simulink model "systema"  (Simulink 7.4)
settings: Solver=ode1  StartTime=0.0  StopTime=1  FixedStep=0.01  RelTol=1e-3
libraries: simulink x7, instrumentlib x2
CloseFcn:
  | rtwprivate ssgencode ModelCloseRequest systema
settings Model: Creator=L503823  LastModifiedBy=tweeter  BufferReuse=off
settings DataIOCC: SignalLoggingName=sigsOut
settings OptimizationCC: OptimizeBlockIOStorage=off  BufferReuse=off  EnforceIntegerDowncast=off  ExpressionFolding=off  FoldNonRolledExpr=off  LocalBlockOutputs=off  InitFltsAndDblsToZero=on
settings DebuggingCC: SaveWithParameterizedLinksMsg=none  SignalResolutionControl=TryResolveAllWithWarning  SolverPrmCheckMsg=none  MultiTaskDSMMsg=warning  MultiTaskCondExecSysMsg=none  StrictBusMsg=ErrorLevel1
settings HardwareCC: TargetUnknown=on
settings RTWCC: IncludeERTFirstTime=on
settings CodeAppCC: IgnoreCustomStorageClasses=off
settings GRTTargetCC: TargetFcnLib=ansi_tfl_tmw.mat  ModelReferenceCompliant=off  MatFileLogging=off

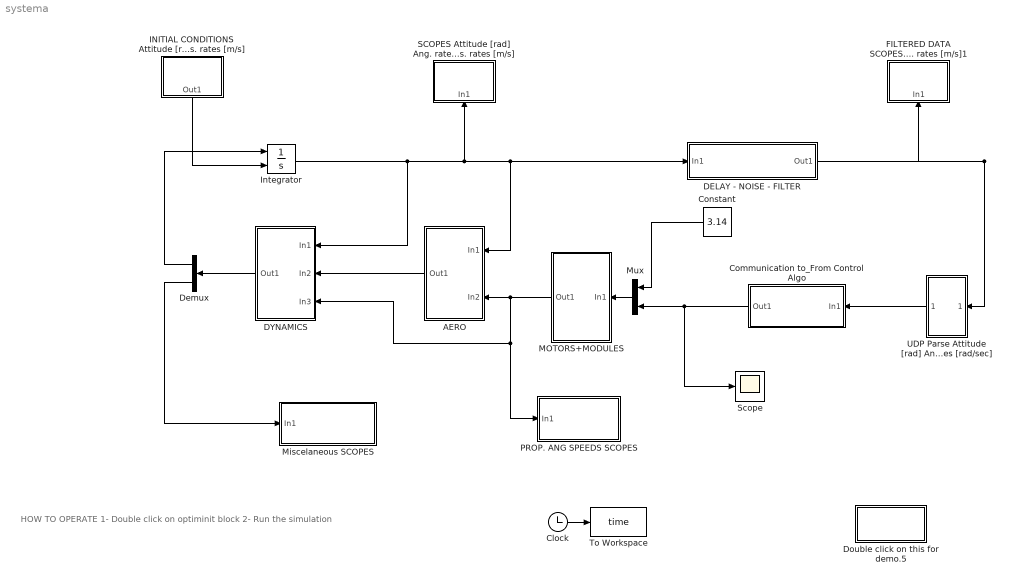
== system systema ==
  note: HOW TO OPERATE
      | 1- Double click on optiminit block
      | 2- Run the simulation
  AERO : Subsystem
  Clock : Clock
      settings: Decimation=10
  Communication to_From Control Algo : Subsystem  TreatAsAtomicUnit=on  SystemSampleTime=.01
  Constant : Constant  Value=3.14  OutDataTypeMode=double  OutDataType=fixdt(1, 16)  OutScaling=2^0  OutDataTypeStr=double  SampleTime=-1
  DELAY - NOISE - FILTER : Subsystem
  DYNAMICS : Subsystem
  Demux : Demux  Outputs=2
  Double click on this for demo.5 : Subsystem
      settings: OpenFcn=optsiminit
      mask Display: disp('optsiminit')
  FILTERED DATA SCOPES Attitude [rad] Ang. rates [rad/sec] position [m] Pos. rates [m/s]1 : Subsystem
  "INITIAL CONDITIONS Attitude [rad] Ang. rates [rad/sec] position [m] Pos. rates [m/s] " : Subsystem
  Integrator : Integrator  InitialConditionSource=external
  MOTORS+MODULES : Subsystem
  Miscelaneous SCOPES : Subsystem
  Mux : Mux  Inputs=2
  PROP. ANG SPEEDS SCOPES : Subsystem
  SCOPES Attitude [rad] Ang. rates [rad/sec] position [m] Pos. rates [m/s] : Subsystem
  Scope : Scope
      settings: YMin=-7.5e+06  YMax=1.25e+07  SaveName=ScopeData11
  To Workspace : ToWorkspace  VariableName=time  SampleTime=-1  SaveFormat=Array
  UDP Parse Attitude [rad] Ang. rates [rad/sec] : Subsystem  TreatAsAtomicUnit=on  SystemSampleTime=.01
  wires:
  Integrator/1 -> DYNAMICS/1(In1), AERO/1(In1), DELAY - NOISE - FILTER/1(In1), SCOPES Attitude [rad] Ang. rates [rad/sec] position [m] Pos. rates [m/s]/1(In1)
  "INITIAL CONDITIONS Attitude [rad] Ang. rates [rad/sec] position [m] Pos. rates [m/s] "/1(Out1) -> Integrator/2
  Clock/1 -> To Workspace/1
  DYNAMICS/1(Out1) -> Demux/1
  Demux/1 -> Integrator/1
  Demux/2 -> Miscelaneous SCOPES/1(In1)
  MOTORS+MODULES/1(Out1) -> AERO/2(In2), DYNAMICS/3(In3), PROP. ANG SPEEDS SCOPES/1(In1)
  AERO/1(Out1) -> DYNAMICS/2(In2)
  DELAY - NOISE - FILTER/1(Out1) -> FILTERED DATA SCOPES Attitude [rad] Ang. rates [rad/sec] position [m] Pos. rates [m/s]1/1(In1), UDP Parse Attitude [rad] Ang. rates [rad/sec]/1(In1)
  UDP Parse Attitude [rad] Ang. rates [rad/sec]/1(Out1) -> Communication to_From Control Algo/1(In1)
  Mux/1 -> MOTORS+MODULES/1(In1)
  Constant/1 -> Mux/1
  Communication to_From Control Algo/1(Out1) -> Mux/2, Scope/1

== system systema/AERO ==
  In1 : Inport  OutDataType=sfix(16)  OutScaling=2^0
  In2 : Inport  Port=2  OutDataType=sfix(16)  OutScaling=2^0
  AERO Attitude [rad] : MATLABFcn  MATLABFcn=aero  OutputDimensions=24
  Mux1 : Mux  Inputs=2
  Out1 : Outport  OutDataType=sfix(16)  OutScaling=2^0
  wires:
  In1/1 -> Mux1/1
  In2/1 -> Mux1/2
  Mux1/1 -> AERO Attitude [rad]/1
  AERO Attitude [rad]/1 -> Out1/1

== system systema/Communication to_From Control Algo ==
  In1 : Inport  OutDataType=fixdt(1, 16)  OutScaling=2^0
  UDP Receive : instrumentlib/UDP Receive  Priority=2  DialogController=instrumentcreatedialog  DialogControllerArgs=DataTag0  Host=127.0.0.1  Port=2500  LocalPort=2500  DataSize="[3  1]"  EnableBlockingMode=on  Timeout=5  SampleTime=-1  DataType=double  ByteOrder=LittleEndian
  UDP Send : instrumentlib/UDP Send  Priority=1  DialogController=instrumentcreatedialog  DialogControllerArgs=DataTag1  Host=127.0.0.1  Port=2040  LocalPort=2041  EnableBlockingMode=on  ByteOrder=LittleEndian
  Out1 : Outport  OutDataType=fixdt(1, 16)  OutScaling=2^0
  wires:
  UDP Receive/1 -> Out1/1
  In1/1 -> UDP Send/1

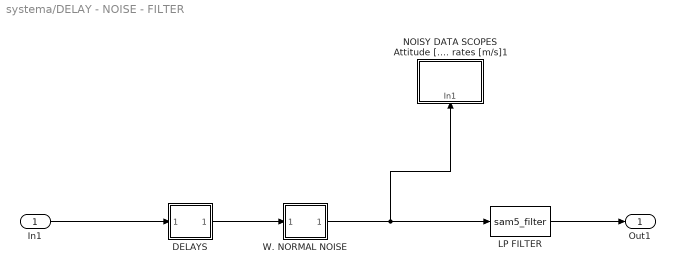
== system systema/DELAY - NOISE - FILTER ==
  In1 : Inport  OutDataType=sfix(16)  OutScaling=2^0
  DELAYS : Subsystem
  LP FILTER : MATLABFcn  MATLABFcn=sam5_filter  OutputDimensions=12  OutputSignalType=real
  NOISY DATA SCOPES Attitude [rad] Ang. rates [rad/sec] position [m] Pos. rates [m/s]1 : Subsystem
  W. NORMAL NOISE : Subsystem
  Out1 : Outport  OutDataType=sfix(16)  OutScaling=2^0
  wires:
  In1/1 -> DELAYS/1(In1)
  DELAYS/1(Out1) -> W. NORMAL NOISE/1(In1)
  W. NORMAL NOISE/1(Out1) -> NOISY DATA SCOPES Attitude [rad] Ang. rates [rad/sec] position [m] Pos. rates [m/s]1/1(In1), LP FILTER/1
  LP FILTER/1 -> Out1/1

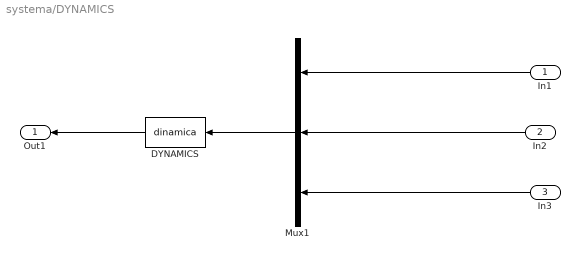
== system systema/DYNAMICS ==
  In1 : Inport  OutDataType=sfix(16)  OutScaling=2^0
  In2 : Inport  Port=2  OutDataType=sfix(16)  OutScaling=2^0
  In3 : Inport  Port=3  OutDataType=sfix(16)  OutScaling=2^0
  DYNAMICS : MATLABFcn  MATLABFcn=dinamica  OutputDimensions=18
  Mux1 : Mux  Inputs=3
  Out1 : Outport  OutDataType=sfix(16)  OutScaling=2^0
  wires:
  DYNAMICS/1 -> Out1/1
  Mux1/1 -> DYNAMICS/1
  In2/1 -> Mux1/2
  In1/1 -> Mux1/1
  In3/1 -> Mux1/3

== system systema/Double click on this for demo.5 ==

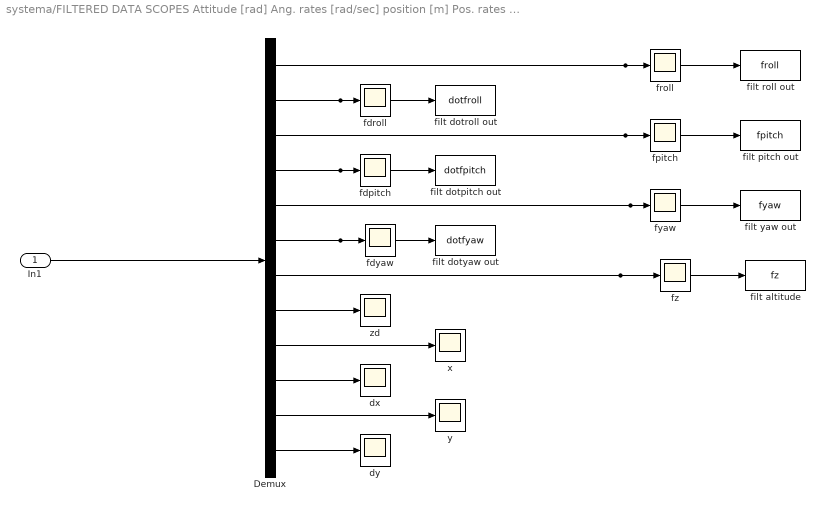
== system systema/FILTERED DATA SCOPES Attitude [rad] Ang. rates [rad/sec] position [m] Pos. rates [m/s]1 ==
  In1 : Inport  OutDataType=sfix(16)  OutScaling=2^0
  Demux : Demux  Outputs=12
  dx : Scope
      settings: TimeRange=5  YMin=0  YMax=0.009  SaveName=ScopeData5
  dy : Scope
      settings: TimeRange=5  YMin=0  YMax=0.009  SaveName=ScopeData10
  fdpitch : Scope
      settings: YMin=-2250  YMax=2250  SaveName=ScopeData15
  fdroll : Scope
      settings: YMin=-0.25  YMax=-0.05  SaveName=ScopeData14
  fdyaw : Scope
      settings: TimeRange=18  YMin=-200  YMax=200  SaveName=ScopeData16
  filt altitude : ToWorkspace  VariableName=fz  SampleTime=-1  SaveFormat=Array
  filt dotpitch out : ToWorkspace  VariableName=dotfpitch  SampleTime=-1  SaveFormat=Array
  filt dotroll out : ToWorkspace  VariableName=dotfroll  SampleTime=-1  SaveFormat=Array
  filt dotyaw out : ToWorkspace  VariableName=dotfyaw  SampleTime=-1  SaveFormat=Array
  filt pitch out : ToWorkspace  VariableName=fpitch  SampleTime=-1  SaveFormat=Array
  filt roll out : ToWorkspace  VariableName=froll  SampleTime=-1  SaveFormat=Array
  filt yaw out : ToWorkspace  VariableName=fyaw  SampleTime=-1  SaveFormat=Array
  fpitch : Scope
      settings: TimeRange=4  YMin=-1  YMax=1
  froll : Scope
      settings: TimeRange=0.25  YMin=-1  YMax=1
  fyaw : Scope
      settings: TimeRange=5  YMin=0  YMax=0.22  SaveName=ScopeData2
  fz : Scope
      settings: TimeRange=5  YMin=-0.45  YMax=0.5  SaveName=ScopeData17
  x : Scope
      settings: TimeRange=5  YMin=0  YMax=0.009  SaveName=ScopeData4
  y : Scope
      settings: TimeRange=5  YMin=0  YMax=0.009  SaveName=ScopeData6
  zd : Scope
      settings: TimeRange=10  YMin=-110.5  YMax=-107.25  SaveName=ScopeData18
  wires:
  Demux/1 -> filt roll out/1, froll/1
  Demux/4 -> fdpitch/1, filt dotpitch out/1
  Demux/8 -> zd/1
  Demux/7 -> filt altitude/1, fz/1
  Demux/6 -> fdyaw/1, filt dotyaw out/1
  Demux/2 -> fdroll/1, filt dotroll out/1
  Demux/5 -> filt yaw out/1, fyaw/1
  Demux/3 -> filt pitch out/1, fpitch/1
  In1/1 -> Demux/1
  Demux/9 -> x/1
  Demux/10 -> dx/1
  Demux/11 -> y/1
  Demux/12 -> dy/1

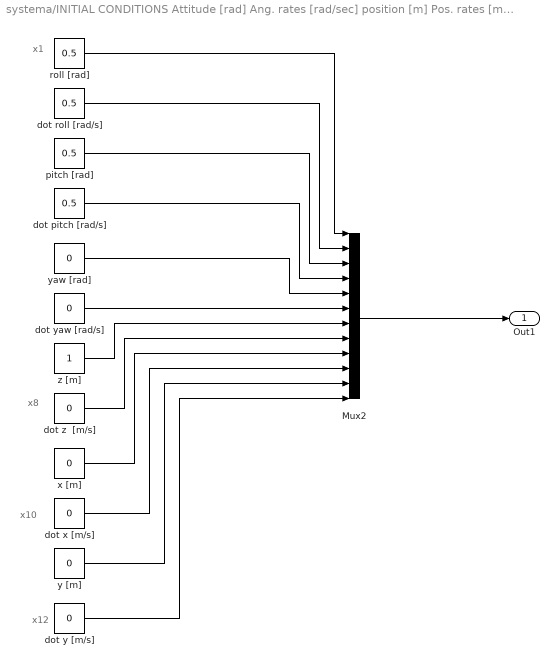
== system systema/INITIAL CONDITIONS Attitude [rad] Ang. rates [rad/sec] position [m] Pos. rates [m/s]  ==
  note: x1
  note: x12
  note: x10
  note: x8
  Mux2 : Mux  Inputs=12
  dot pitch [rad/s] : Constant  Value=0.5  OutDataType=sfix(16)  OutScaling=2^0
  dot roll [rad/s] : Constant  Value=0.5  OutDataType=sfix(16)  OutScaling=2^0
  dot x [m/s] : Constant  Value=0  OutDataType=sfix(16)  OutScaling=2^0
  dot y [m/s] : Constant  Value=0  OutDataType=sfix(16)  OutScaling=2^0
  dot yaw [rad/s] : Constant  Value=0  OutDataType=sfix(16)  OutScaling=2^0
  dot z  [m/s] : Constant  Value=0  OutDataType=sfix(16)  OutScaling=2^0
  pitch [rad] : Constant  Value=0.5  OutDataType=sfix(16)  OutScaling=2^0
  roll [rad] : Constant  Value=0.5  OutDataType=sfix(16)  OutScaling=2^0
  x [m] : Constant  Value=0  OutDataType=sfix(16)  OutScaling=2^0
  y [m] : Constant  Value=0  OutDataType=sfix(16)  OutScaling=2^0
  yaw [rad] : Constant  Value=0  OutDataType=sfix(16)  OutScaling=2^0
  z [m] : Constant  OutDataType=sfix(16)  OutScaling=2^0
  Out1 : Outport  OutDataType=sfix(16)  OutScaling=2^0
  wires:
  roll [rad]/1 -> Mux2/1
  dot roll [rad/s]/1 -> Mux2/2
  pitch [rad]/1 -> Mux2/3
  dot pitch [rad/s]/1 -> Mux2/4
  dot yaw [rad/s]/1 -> Mux2/6
  z [m]/1 -> Mux2/7
  dot z  [m/s]/1 -> Mux2/8
  yaw [rad]/1 -> Mux2/5
  Mux2/1 -> Out1/1
  x [m]/1 -> Mux2/9
  dot x [m/s]/1 -> Mux2/10
  y [m]/1 -> Mux2/11
  dot y [m/s]/1 -> Mux2/12

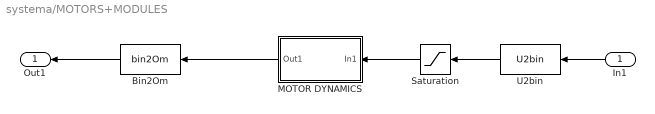
== system systema/MOTORS+MODULES ==
  In1 : Inport  OutDataType=sfix(16)  OutScaling=2^0
  Bin2Om : MATLABFcn  MATLABFcn=bin2Om  OutputDimensions=4  OutputSignalType=real
  MOTOR DYNAMICS : Subsystem
  Saturation : Saturate  UpperLimit=125  LowerLimit=10
  U2bin : MATLABFcn  MATLABFcn=U2bin  OutputDimensions=4  OutputSignalType=real
  Out1 : Outport  OutDataType=sfix(16)  OutScaling=2^0
  wires:
  Bin2Om/1 -> Out1/1
  MOTOR DYNAMICS/1(Out1) -> Bin2Om/1
  U2bin/1 -> Saturation/1
  In1/1 -> U2bin/1
  Saturation/1 -> MOTOR DYNAMICS/1(In1)

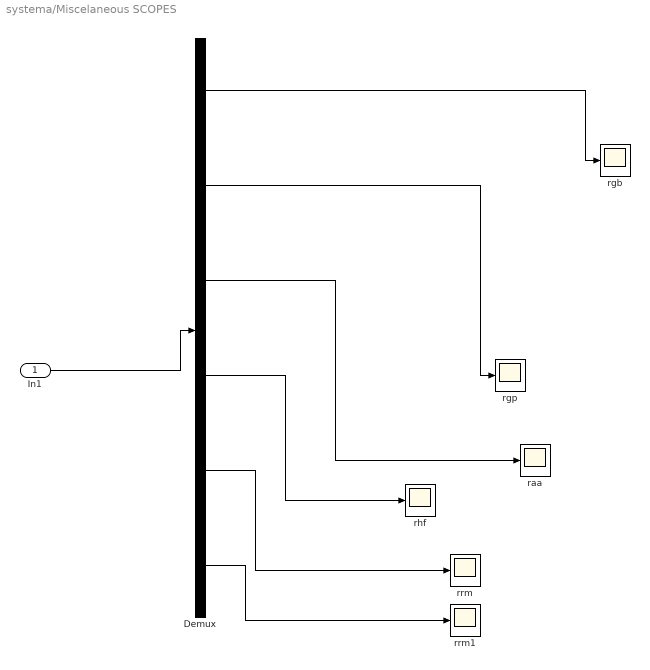
== system systema/Miscelaneous SCOPES ==
  In1 : Inport  PortDimensions=6  OutDataType=sfix(16)  OutScaling=2^0
  Demux : Demux  Outputs=6
  raa : Scope
      settings: TimeRange=18  YMin=-200  YMax=200  SaveName=ScopeData16
  rgb : Scope
      settings: YMin=-0.25  YMax=-0.05  SaveName=ScopeData14
  rgp : Scope
      settings: YMin=-2250  YMax=2250  SaveName=ScopeData15
  rhf : Scope
      settings: TimeRange=10  YMin=-110.5  YMax=-107.25  SaveName=ScopeData18
  rrm : Scope
      settings: TimeRange=5  YMin=-4.75e-015  YMax=0  SaveName=ScopeData25
  rrm1 : Scope
      settings: TimeRange=5  YMin=-4.75e-015  YMax=0  SaveName=ScopeData3
  wires:
  In1/1 -> Demux/1
  Demux/5 -> rrm/1
  Demux/4 -> rhf/1
  Demux/3 -> raa/1
  Demux/2 -> rgp/1
  Demux/1 -> rgb/1
  Demux/6 -> rrm1/1

== system systema/PROP. ANG SPEEDS SCOPES ==
  In1 : Inport  OutDataType=sfix(16)  OutScaling=2^0
  Demux1 : Demux
  omega{1..4} (4 alike) : Scope
      omega1 settings: TimeRange=3.5  YMin=144.101  YMax=144.104  SaveName=ScopeData7
      omega2 settings: YMin=142.5  YMax=147.5  SaveName=ScopeData8
      omega3 settings: YMin=0  YMax=150  SaveName=ScopeData9
      omega4 settings: YMin=0  YMax=150  SaveName=ScopeData14
  wires:
  Demux1/1 -> omega1/1
  Demux1/2 -> omega2/1
  Demux1/3 -> omega3/1
  Demux1/4 -> omega4/1
  In1/1 -> Demux1/1

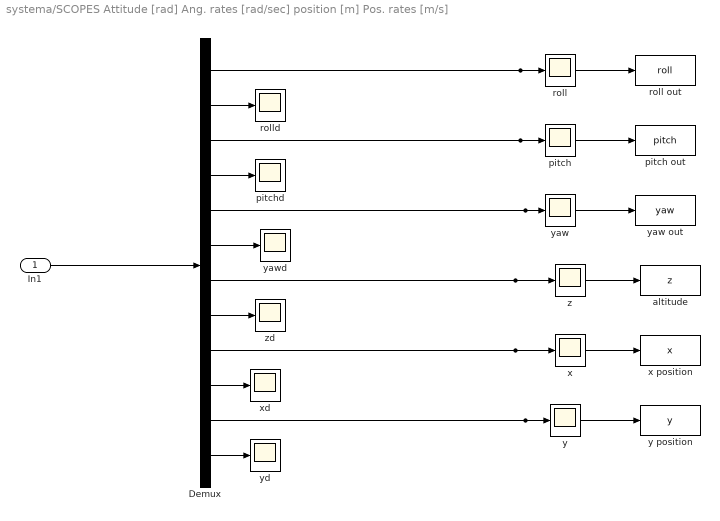
== system systema/SCOPES Attitude [rad] Ang. rates [rad/sec] position [m] Pos. rates [m/s] ==
  In1 : Inport  OutDataType=sfix(16)  OutScaling=2^0
  Demux : Demux  Outputs=12
  altitude : ToWorkspace  VariableName=z  SampleTime=-1  SaveFormat=Array
  pitch : Scope
      settings: TimeRange=4  YMin=-0.08  YMax=0.16
  pitch out : ToWorkspace  VariableName=pitch  SampleTime=-1  SaveFormat=Array
  pitchd : Scope
      settings: YMin=-1.75  YMax=1.75  SaveName=ScopeData15
  roll : Scope
      settings: TimeRange=0.25  YMin=-0.008  YMax=0.005
  roll out : ToWorkspace  VariableName=roll  SampleTime=-1  SaveFormat=Array
  rolld : Scope
      settings: TimeRange=7  YMin=-0.15  YMax=0.125  SaveName=ScopeData14
  x : Scope
      settings: TimeRange=5  YMin=-1  YMax=1  SaveName=ScopeData24
  x position : ToWorkspace  VariableName=x  SampleTime=-1  SaveFormat=Array
  xd : Scope
      settings: TimeRange=5  YMin=-4.75e-015  YMax=0  SaveName=ScopeData25
  y : Scope
      settings: TimeRange=5  YMin=-1  YMax=1  SaveName=ScopeData26
  y position : ToWorkspace  VariableName=y  SampleTime=-1  SaveFormat=Array
  yaw : Scope
      settings: TimeRange=5  YMin=-175  YMax=0  SaveName=ScopeData2
  yaw out : ToWorkspace  VariableName=yaw  SampleTime=-1  SaveFormat=Array
  yawd : Scope
      settings: TimeRange=18  YMin=-0.275  YMax=0.15  SaveName=ScopeData16
  yd : Scope
      settings: TimeRange=5  YMin=-143.75  YMax=-141.75  SaveName=ScopeData27
  z : Scope
      settings: TimeRange=5  YMin=0  YMax=0.009  SaveName=ScopeData17
  zd : Scope
      settings: TimeRange=10  YMin=-110.5  YMax=-107.25  SaveName=ScopeData18
  wires:
  In1/1 -> Demux/1
  Demux/3 -> pitch/1, pitch out/1
  Demux/5 -> yaw/1, yaw out/1
  Demux/2 -> rolld/1
  Demux/6 -> yawd/1
  Demux/7 -> z/1, altitude/1
  Demux/8 -> zd/1
  Demux/9 -> x/1, x position/1
  Demux/11 -> y/1, y position/1
  Demux/12 -> yd/1
  Demux/10 -> xd/1
  Demux/4 -> pitchd/1
  Demux/1 -> roll/1, roll out/1

== system systema/UDP Parse Attitude [rad] Ang. rates [rad/sec] ==
  In1 : Inport  OutDataType=sfix(16)  OutScaling=2^0
  Demux : Demux  Outputs=12
  Mux : Mux  Inputs=6
  Out1 : Outport  OutDataType=sfix(16)  OutScaling=2^0
  wires:
  Demux/1 -> Mux/1
  Demux/3 -> Mux/2
  Demux/5 -> Mux/3
  Demux/2 -> Mux/4
  Demux/4 -> Mux/5
  Demux/6 -> Mux/6
  In1/1 -> Demux/1
  Mux/1 -> Out1/1

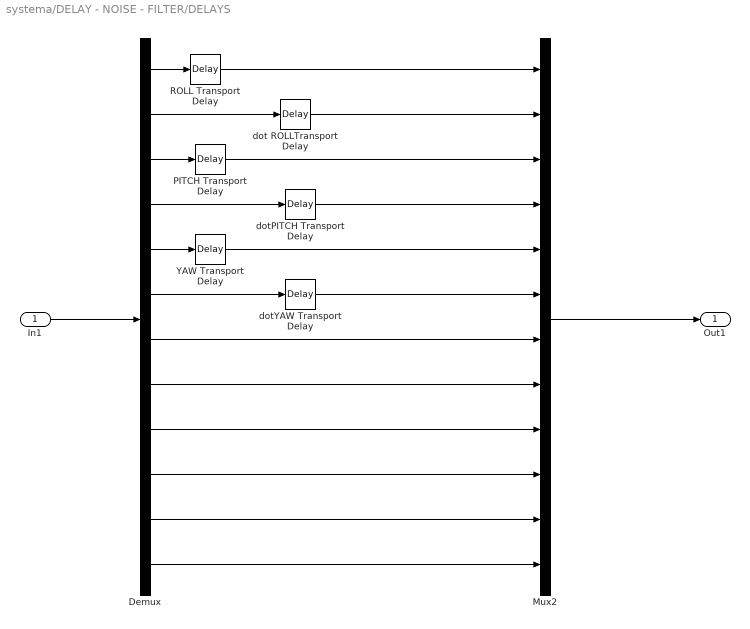
== system systema/DELAY - NOISE - FILTER/DELAYS ==
  In1 : Inport  OutDataType=sfix(16)  OutScaling=2^0
  Demux : Demux  Outputs=12
  Mux2 : Mux  Inputs=12
  PITCH Transport Delay : TransportDelay  DelayTime=8E-3
  ROLL Transport Delay : TransportDelay  DelayTime=8E-3
  YAW Transport Delay : TransportDelay  DelayTime=8E-3
  dot ROLLTransport Delay : TransportDelay  DelayTime=4.5E-3
  dotPITCH Transport Delay : TransportDelay  DelayTime=4.5E-3
  dotYAW Transport Delay : TransportDelay  DelayTime=4.5E-3
  Out1 : Outport  OutDataType=sfix(16)  OutScaling=2^0
  wires:
  dot ROLLTransport Delay/1 -> Mux2/2
  Demux/12 -> Mux2/12
  Demux/11 -> Mux2/11
  Demux/10 -> Mux2/10
  Demux/9 -> Mux2/9
  Demux/8 -> Mux2/8
  Demux/7 -> Mux2/7
  dotYAW Transport Delay/1 -> Mux2/6
  Demux/6 -> dotYAW Transport Delay/1
  YAW Transport Delay/1 -> Mux2/5
  Demux/5 -> YAW Transport Delay/1
  dotPITCH Transport Delay/1 -> Mux2/4
  Demux/4 -> dotPITCH Transport Delay/1
  PITCH Transport Delay/1 -> Mux2/3
  Demux/3 -> PITCH Transport Delay/1
  Demux/2 -> dot ROLLTransport Delay/1
  ROLL Transport Delay/1 -> Mux2/1
  Demux/1 -> ROLL Transport Delay/1
  In1/1 -> Demux/1
  Mux2/1 -> Out1/1

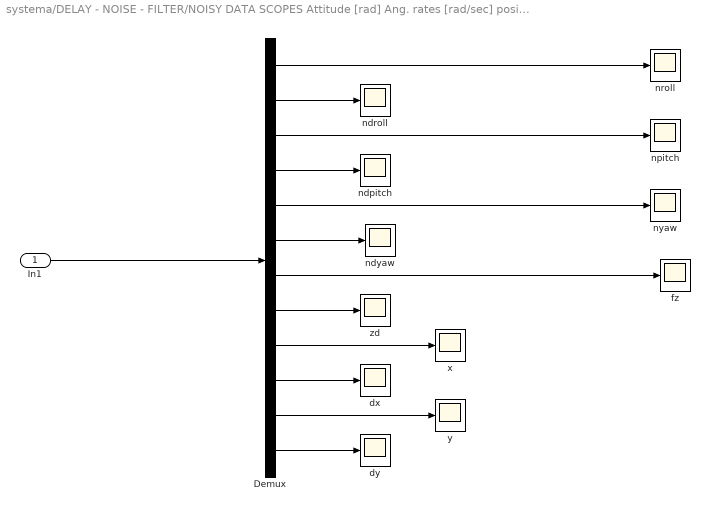
== system systema/DELAY - NOISE - FILTER/NOISY DATA SCOPES Attitude [rad] Ang. rates [rad/sec] position [m] Pos. rates [m/s]1 ==
  In1 : Inport  OutDataType=sfix(16)  OutScaling=2^0
  Demux : Demux  Outputs=12
  dx : Scope
      settings: TimeRange=5  YMin=0  YMax=0.009  SaveName=ScopeData5
  dy : Scope
      settings: TimeRange=5  YMin=0  YMax=0.009  SaveName=ScopeData10
  fz : Scope
      settings: TimeRange=5  YMin=0  YMax=0.009  SaveName=ScopeData17
  ndpitch : Scope
      settings: YMin=-2250  YMax=2250  SaveName=ScopeData15
  ndroll : Scope
      settings: YMin=-0.25  YMax=-0.05  SaveName=ScopeData14
  ndyaw : Scope
      settings: TimeRange=18  YMin=-200  YMax=200  SaveName=ScopeData16
  npitch : Scope
      settings: TimeRange=4  YMin=-1  YMax=1
  nroll : Scope
      settings: TimeRange=0.25  YMin=-1  YMax=1
  nyaw : Scope
      settings: TimeRange=5  YMin=0  YMax=0.22  SaveName=ScopeData2
  x : Scope
      settings: TimeRange=5  YMin=0  YMax=0.009  SaveName=ScopeData4
  y : Scope
      settings: TimeRange=5  YMin=0  YMax=0.009  SaveName=ScopeData6
  zd : Scope
      settings: TimeRange=10  YMin=-110.5  YMax=-107.25  SaveName=ScopeData18
  wires:
  Demux/1 -> nroll/1
  Demux/4 -> ndpitch/1
  Demux/8 -> zd/1
  Demux/7 -> fz/1
  Demux/6 -> ndyaw/1
  Demux/2 -> ndroll/1
  Demux/5 -> nyaw/1
  Demux/3 -> npitch/1
  In1/1 -> Demux/1
  Demux/9 -> x/1
  Demux/10 -> dx/1
  Demux/11 -> y/1
  Demux/12 -> dy/1

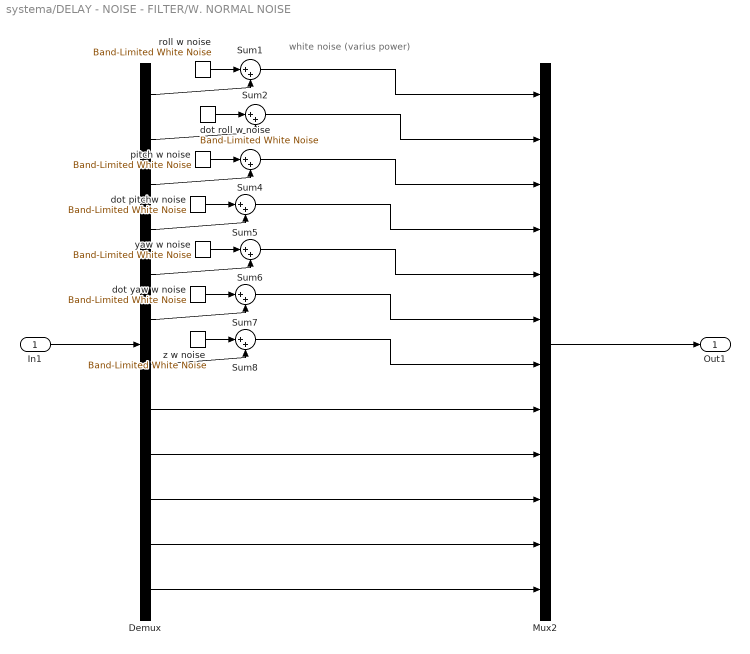
== system systema/DELAY - NOISE - FILTER/W. NORMAL NOISE ==
  note: white noise (varius power)
  In1 : Inport  OutDataType=sfix(16)  OutScaling=2^0
  Demux : Demux  Outputs=12
  Mux2 : Mux  Inputs=12
  Sum{1..2,4..8} (7 alike) : Sum  Inputs=|++  OutDataType=sfix(16)  OutScaling=2^0  SaturateOnIntegerOverflow=on
  dot pitchw noise : simulink/Sources/Band-Limited White Noise  SystemSampleTime=-1  Cov=[0.0001]  Ts=0.01  seed=[23341]
  dot roll w noise : simulink/Sources/Band-Limited White Noise  SystemSampleTime=-1  Cov=[0.0001]  Ts=0.01  seed=[23341]
  dot yaw w noise : simulink/Sources/Band-Limited White Noise  SystemSampleTime=-1  Cov=[0.0001]  Ts=0.01  seed=[23341]
  pitch w noise : simulink/Sources/Band-Limited White Noise  SystemSampleTime=-1  Cov=[0.00001]  Ts=0.01  seed=[23341]
  roll w noise : simulink/Sources/Band-Limited White Noise  SystemSampleTime=-1  Cov=[0.00001]  Ts=0.01  seed=[24431]
  yaw w noise : simulink/Sources/Band-Limited White Noise  SystemSampleTime=-1  Cov=[0.00001]  Ts=0.01  seed=[23341]
  z w noise : simulink/Sources/Band-Limited White Noise  SystemSampleTime=-1  Cov=[0.00001]  Ts=0.01  seed=[23341]
  Out1 : Outport  OutDataType=sfix(16)  OutScaling=2^0
  wires:
  Demux/8 -> Mux2/8
  Demux/12 -> Mux2/12
  Demux/11 -> Mux2/11
  Demux/10 -> Mux2/10
  Demux/9 -> Mux2/9
  Sum8/1 -> Mux2/7
  z w noise/1 -> Sum8/1
  Demux/7 -> Sum8/2
  Sum7/1 -> Mux2/6
  dot yaw w noise/1 -> Sum7/1
  Demux/6 -> Sum7/2
  Sum6/1 -> Mux2/5
  yaw w noise/1 -> Sum6/1
  Demux/5 -> Sum6/2
  Sum5/1 -> Mux2/4
  dot pitchw noise/1 -> Sum5/1
  Demux/4 -> Sum5/2
  Sum4/1 -> Mux2/3
  pitch w noise/1 -> Sum4/1
  Demux/3 -> Sum4/2
  Sum2/1 -> Mux2/2
  dot roll w noise/1 -> Sum2/1
  Demux/2 -> Sum2/2
  Sum1/1 -> Mux2/1
  roll w noise/1 -> Sum1/1
  Mux2/1 -> Out1/1
  In1/1 -> Demux/1
  Demux/1 -> Sum1/2

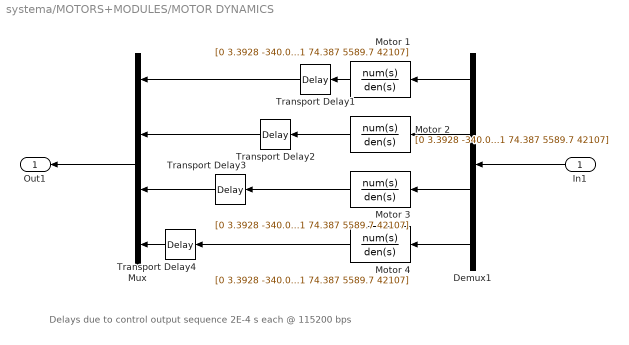
== system systema/MOTORS+MODULES/MOTOR DYNAMICS ==
  note: Delays due to control output sequence
      | 2E-4 s each @ 115200 bps
  In1 : Inport  OutDataType=sfix(16)  OutScaling=2^0
  Demux1 : Demux
  Motor {1..4} (4 alike) : TransferFcn  Numerator=[0 3.3928 -340.09 39451]  Denominator=[1 74.387 5589.7 42107]
  Mux : Mux
  Transport Delay1 : TransportDelay  DelayTime=2E-4
  Transport Delay2 : TransportDelay  DelayTime=4E-4
  Transport Delay3 : TransportDelay  DelayTime=6E-4
  Transport Delay4 : TransportDelay  DelayTime=8E-4
  Out1 : Outport  OutDataType=sfix(16)  OutScaling=2^0
  wires:
  In1/1 -> Demux1/1
  Demux1/1 -> Motor 1/1
  Demux1/2 -> Motor 2/1
  Demux1/3 -> Motor 3/1
  Demux1/4 -> Motor 4/1
  Motor 1/1 -> Transport Delay1/1
  Motor 2/1 -> Transport Delay2/1
  Motor 3/1 -> Transport Delay3/1
  Motor 4/1 -> Transport Delay4/1
  Mux/1 -> Out1/1
  Transport Delay2/1 -> Mux/2
  Transport Delay3/1 -> Mux/3
  Transport Delay4/1 -> Mux/4
  Transport Delay1/1 -> Mux/1
